simulink model "IEEE14_case"  (R2024b)
settings: Solver=FixedStepAuto  StartTime=0  StopTime=2  FixedStep=1e-7  RelTol=1e-3
values from neighbouring files (symbols this model uses):
  GFL_15_Bva = 0.009    [IEEE14_parameters.m]
  GFL_15_C_bus_pu = 7.179419    [IEEE14_parameters.m]
  GFL_15_f0 = 60    [IEEE14_parameters.m]
  GFL_15_I_id = 691.26967    [IEEE14_parameters.m]
  GFL_15_I_iq = 691.26967    [IEEE14_parameters.m]
  GFL_15_I_od = 45.2207    [IEEE14_parameters.m]
  GFL_15_I_oq = 45.2207    [IEEE14_parameters.m]
  GFL_15_I_pll = 0.78    [IEEE14_parameters.m]
  GFL_15_Kdi = 0.09    [IEEE14_parameters.m]
  GFL_15_Kdo = 0.9    [IEEE14_parameters.m]
  GFL_15_Kqi = 0.09    [IEEE14_parameters.m]
  GFL_15_Kqo = 0.9    [IEEE14_parameters.m]
  GFL_15_Lg_pu = 0.631447    [IEEE14_parameters.m]
  GFL_15_mode = 1    [IEEE14_parameters.m]
  GFL_15_P_id = 3.7166    [IEEE14_parameters.m]
  GFL_15_P_iq = 3.7166    [IEEE14_parameters.m]
  GFL_15_P_od = 0.4798    [IEEE14_parameters.m]
  GFL_15_P_oq = 0.4798    [IEEE14_parameters.m]
  GFL_15_P_pll = 290.42    [IEEE14_parameters.m]
  GFL_15_Qe_ref = 0.2    [IEEE14_parameters.m]
  GFL_15_Rg_pu = 0.024016    [IEEE14_parameters.m]
  GFL_15_Sbase = 1.000000e+4    (= 10000)    [IEEE14_parameters.m]
  GFL_15_Tdi = 0.01    [IEEE14_parameters.m]
  GFL_15_Tdo = 0.2    [IEEE14_parameters.m]
  GFL_15_Tqi = 0.01    [IEEE14_parameters.m]
  GFL_15_Tqo = 0.2    [IEEE14_parameters.m]
  GFL_15_Vbase = 380    [IEEE14_parameters.m]
  GFL_15_Vdc_ref = 1.011475    [IEEE14_parameters.m]
  GFL_15_Vdcbase = 700    [IEEE14_parameters.m]
  GFL_15_vq_ref = 0    [IEEE14_parameters.m]
  GFL_16_Bva = 0.002    [IEEE14_parameters.m]
  GFL_16_C_bus_pu = 7.179419    [IEEE14_parameters.m]
  GFL_16_f0 = 60    [IEEE14_parameters.m]
  GFL_16_I_id = 691.26967    [IEEE14_parameters.m]
  GFL_16_I_iq = 691.26967    [IEEE14_parameters.m]
  GFL_16_I_od = 45.2207    [IEEE14_parameters.m]
  GFL_16_I_oq = 45.2207    [IEEE14_parameters.m]
  GFL_16_I_pll = 0.78    [IEEE14_parameters.m]
  GFL_16_Kdi = 0.05    [IEEE14_parameters.m]
  GFL_16_Kdo = 0.5    [IEEE14_parameters.m]
  GFL_16_Kqi = 0.05    [IEEE14_parameters.m]
  GFL_16_Kqo = 0.5    [IEEE14_parameters.m]
  GFL_16_Lg_pu = 0.631447    [IEEE14_parameters.m]
  GFL_16_mode = 1    [IEEE14_parameters.m]
  GFL_16_P_id = 3.7166    [IEEE14_parameters.m]
  GFL_16_P_iq = 3.7166    [IEEE14_parameters.m]
  GFL_16_P_od = 0.4798    [IEEE14_parameters.m]
  GFL_16_P_oq = 0.4798    [IEEE14_parameters.m]
  GFL_16_P_pll = 290.42    [IEEE14_parameters.m]
  GFL_16_Qe_ref = 0.2    [IEEE14_parameters.m]
  GFL_16_Rg_pu = 0.024016    [IEEE14_parameters.m]
  GFL_16_Sbase = 1.000000e+4    (= 10000)    [IEEE14_parameters.m]
  GFL_16_Tdi = 0.01    [IEEE14_parameters.m]
  GFL_16_Tdo = 0.2    [IEEE14_parameters.m]
  GFL_16_Tqi = 0.01    [IEEE14_parameters.m]
  GFL_16_Tqo = 0.2    [IEEE14_parameters.m]
  GFL_16_Vbase = 380    [IEEE14_parameters.m]
  GFL_16_Vdc_ref = 1.01144    [IEEE14_parameters.m]
  GFL_16_Vdcbase = 700    [IEEE14_parameters.m]
  GFL_16_vq_ref = 0    [IEEE14_parameters.m]
  GFL_17_Bva = 0.002    [IEEE14_parameters.m]
  GFL_17_C_bus_pu = 7.179419    [IEEE14_parameters.m]
  GFL_17_f0 = 60    [IEEE14_parameters.m]
  GFL_17_I_id = 691.26967    [IEEE14_parameters.m]
  GFL_17_I_iq = 691.26967    [IEEE14_parameters.m]
  GFL_17_I_od = 45.2207    [IEEE14_parameters.m]
  GFL_17_I_oq = 45.2207    [IEEE14_parameters.m]
  GFL_17_I_pll = 0.78    [IEEE14_parameters.m]
  GFL_17_Kdi = 0.05    [IEEE14_parameters.m]
  GFL_17_Kdo = 0.5    [IEEE14_parameters.m]
  GFL_17_Kqi = 0.05    [IEEE14_parameters.m]
  GFL_17_Kqo = 0.5    [IEEE14_parameters.m]
  GFL_17_Lg_pu = 0.631447    [IEEE14_parameters.m]
  GFL_17_mode = 1    [IEEE14_parameters.m]
  GFL_17_P_id = 3.7166    [IEEE14_parameters.m]
  GFL_17_P_iq = 3.7166    [IEEE14_parameters.m]
  GFL_17_P_od = 0.4798    [IEEE14_parameters.m]
  GFL_17_P_oq = 0.4798    [IEEE14_parameters.m]
  GFL_17_P_pll = 290.42    [IEEE14_parameters.m]
  GFL_17_Qe_ref = 0.2    [IEEE14_parameters.m]
  GFL_17_Rg_pu = 0.024016    [IEEE14_parameters.m]
  GFL_17_Sbase = 1.000000e+4    (= 10000)    [IEEE14_parameters.m]
  GFL_17_Tdi = 0.01    [IEEE14_parameters.m]
  GFL_17_Tdo = 0.2    [IEEE14_parameters.m]
  GFL_17_Tqi = 0.01    [IEEE14_parameters.m]
  GFL_17_Tqo = 0.2    [IEEE14_parameters.m]
  GFL_17_Vbase = 380    [IEEE14_parameters.m]
  GFL_17_Vdc_ref = 1.011632    [IEEE14_parameters.m]
  GFL_17_Vdcbase = 700    [IEEE14_parameters.m]
  GFL_17_vq_ref = 0    [IEEE14_parameters.m]
  GFL_18_Bva = 0.002    [IEEE14_parameters.m]
  GFL_18_C_bus_pu = 7.179419    [IEEE14_parameters.m]
  GFL_18_f0 = 60    [IEEE14_parameters.m]
  GFL_18_I_id = 691.26967    [IEEE14_parameters.m]
  GFL_18_I_iq = 691.26967    [IEEE14_parameters.m]
  GFL_18_I_od = 45.2207    [IEEE14_parameters.m]
  GFL_18_I_oq = 45.2207    [IEEE14_parameters.m]
  GFL_18_I_pll = 0.78    [IEEE14_parameters.m]
  GFL_18_Kdi = 0.05    [IEEE14_parameters.m]
  GFL_18_Kdo = 0.5    [IEEE14_parameters.m]
  GFL_18_Kqi = 0.05    [IEEE14_parameters.m]
  GFL_18_Kqo = 0.5    [IEEE14_parameters.m]
  GFL_18_Lg_pu = 0.631447    [IEEE14_parameters.m]
  GFL_18_mode = 1    [IEEE14_parameters.m]
  GFL_18_P_id = 3.7166    [IEEE14_parameters.m]
  GFL_18_P_iq = 3.7166    [IEEE14_parameters.m]
  GFL_18_P_od = 0.4798    [IEEE14_parameters.m]
  GFL_18_P_oq = 0.4798    [IEEE14_parameters.m]
  GFL_18_P_pll = 290.42    [IEEE14_parameters.m]
  GFL_18_Qe_ref = 0.2    [IEEE14_parameters.m]
  GFL_18_Rg_pu = 0.024016    [IEEE14_parameters.m]
  GFL_18_Sbase = 1.000000e+4    (= 10000)    [IEEE14_parameters.m]
  GFL_18_Tdi = 0.01    [IEEE14_parameters.m]
  GFL_18_Tdo = 0.2    [IEEE14_parameters.m]
  GFL_18_Tqi = 0.01    [IEEE14_parameters.m]
  GFL_18_Tqo = 0.2    [IEEE14_parameters.m]
  GFL_18_Vbase = 380    [IEEE14_parameters.m]
  GFL_18_Vdc_ref = 1.011572    [IEEE14_parameters.m]
  GFL_18_Vdcbase = 700    [IEEE14_parameters.m]
  GFL_18_vq_ref = 0    [IEEE14_parameters.m]
  ... (+180 more)
(part 3 of 25)

== system IEEE14_case/GFL_15 ==
  v_d_GFL_15 : Inport
  v_q_GFL_15 : Inport  Port=2
  i_dc_GFL_15 : Inport  Port=3
  Idv_GFL_15 : Integrator  InitialCondition=-9.005176619289375e-21
  Iqv_GFL_15 : Integrator  InitialCondition=212.99246240000113
  Phi_ga_GFL_15 : Integrator  InitialCondition=14.405272691494698
  Phi_gb_GFL_15 : Integrator  InitialCondition=4.700156753170725
  Phi_gc_GFL_15 : Integrator  InitialCondition=-215.7031229683803
  Phi_gd_GFL_15 : Integrator  InitialCondition=-0.9400313506342463
  Phipll_GFL_15 : Integrator  InitialCondition=-8.990901410054388e-21
  Psi_d_GFL_15 : Integrator  InitialCondition=1.758329914032016e-21
  Psi_q_GFL_15 : Integrator  InitialCondition=21.299246240000112
  V_dc_GFL_15 : Integrator  InitialCondition=708.0324770006274
  d_Idv_GFL_15_block : Subsystem
  d_Iqv_GFL_15_block : Subsystem
  d_Phi_ga_GFL_15_block : Subsystem
  d_Phi_gb_GFL_15_block : Subsystem
  d_Phi_gc_GFL_15_block : Subsystem
  d_Phi_gd_GFL_15_block : Subsystem
  d_Phipll_GFL_15_block : Subsystem
  d_Psi_d_GFL_15_block : Subsystem
  d_Psi_q_GFL_15_block : Subsystem
  d_V_dc_GFL_15_block : Subsystem
  d_i_gd_GFL_15_block : Subsystem
  d_i_gq_GFL_15_block : Subsystem
  d_theta_pll_GFL_15_block : Subsystem
  e_dc_GFL_15_block : Subsystem
  i_d_GFL_15_block : Subsystem
  i_gd_GFL_15 : Integrator  InitialCondition=13.553302841894695
  i_gq_GFL_15 : Integrator  InitialCondition=-2.710660568379226
  i_q_GFL_15_block : Subsystem
  theta_pll_GFL_15 : Integrator  InitialCondition=0.12960466832124
  i_d_GFL_15 : Outport
  i_q_GFL_15 : Outport  Port=2
  e_dc_GFL_15 : Outport  Port=3
  wires:
  V_dc_GFL_15/1 -> d_V_dc_GFL_15_block/1(State_V_dc_GFL_15_d284c), d_V_dc_GFL_15_block/10(State_V_dc_GFL_15_e0213), d_V_dc_GFL_15_block/42(State_V_dc_GFL_15_5df59), d_i_gd_GFL_15_block/6(State_V_dc_GFL_15_5ead9), d_Phi_gb_GFL_15_block/6(State_V_dc_GFL_15_cf545), d_Phi_ga_GFL_15_block/1(State_V_dc_GFL_15_371a8), e_dc_GFL_15_block/1(State_V_dc_GFL_15_93b67)
  theta_pll_GFL_15/1 -> d_i_gq_GFL_15_block/10(State_theta_pll_GFL_15_ed7e5), d_i_gq_GFL_15_block/13(State_theta_pll_GFL_15_a894f), d_i_gq_GFL_15_block/15(State_theta_pll_GFL_15_7b0e7), d_V_dc_GFL_15_block/6(State_theta_pll_GFL_15_67f5c), d_i_gq_GFL_15_block/8(State_theta_pll_GFL_15_b231d), d_V_dc_GFL_15_block/8(State_theta_pll_GFL_15_bdd37), d_V_dc_GFL_15_block/15(State_theta_pll_GFL_15_3bef8), d_V_dc_GFL_15_block/17(State_theta_pll_GFL_15_b898b), d_V_dc_GFL_15_block/23(State_theta_pll_GFL_15_82eb1), d_V_dc_GFL_15_block/27(State_theta_pll_GFL_15_9ca51), d_V_dc_GFL_15_block/32(State_theta_pll_GFL_15_ec66b), d_i_gd_GFL_15_block/4(State_theta_pll_GFL_15_781ce), d_V_dc_GFL_15_block/34(State_theta_pll_GFL_15_4b302), d_i_gq_GFL_15_block/2(State_theta_pll_GFL_15_94dd7), d_V_dc_GFL_15_block/41(State_theta_pll_GFL_15_0f1b8), d_theta_pll_GFL_15_block/4(State_theta_pll_GFL_15_f7355), d_Phi_gb_GFL_15_block/2(State_theta_pll_GFL_15_82324), d_Phi_gb_GFL_15_block/4(State_theta_pll_GFL_15_58522), d_V_dc_GFL_15_block/39(State_theta_pll_GFL_15_39e34), d_Phi_gd_GFL_15_block/4(State_theta_pll_GFL_15_d2b83), d_Phi_gd_GFL_15_block/2(State_theta_pll_GFL_15_e398b), d_Phi_gd_GFL_15_block/8(State_theta_pll_GFL_15_37f0e), d_Phi_gd_GFL_15_block/10(State_theta_pll_GFL_15_ae580), d_Phi_gd_GFL_15_block/13(State_theta_pll_GFL_15_e05ad), d_Phi_gd_GFL_15_block/15(State_theta_pll_GFL_15_0e420), d_Idv_GFL_15_block/3(State_theta_pll_GFL_15_12ffd), d_Idv_GFL_15_block/5(State_theta_pll_GFL_15_9725f), d_i_gq_GFL_15_block/4(State_theta_pll_GFL_15_89960), d_Idv_GFL_15_block/9(State_theta_pll_GFL_15_2202b), d_Iqv_GFL_15_block/9(State_theta_pll_GFL_15_f624d), d_V_dc_GFL_15_block/21(State_theta_pll_GFL_15_c9fe8), d_Iqv_GFL_15_block/7(State_theta_pll_GFL_15_e8e0d), d_Iqv_GFL_15_block/3(State_theta_pll_GFL_15_5bce6), d_i_gd_GFL_15_block/2(State_theta_pll_GFL_15_a07ec), d_Iqv_GFL_15_block/5(State_theta_pll_GFL_15_c6881), d_Phipll_GFL_15_block/2(State_theta_pll_GFL_15_65253), d_Phi_gc_GFL_15_block/3(State_theta_pll_GFL_15_5b93f), d_Phi_gc_GFL_15_block/5(State_theta_pll_GFL_15_647bc), d_Phi_gc_GFL_15_block/10(State_theta_pll_GFL_15_159ad), d_Psi_d_GFL_15_block/2(State_theta_pll_GFL_15_95588), d_Psi_d_GFL_15_block/4(State_theta_pll_GFL_15_90724), d_Psi_q_GFL_15_block/2(State_theta_pll_GFL_15_42098), d_Psi_q_GFL_15_block/4(State_theta_pll_GFL_15_5b172), i_d_GFL_15_block/2(State_theta_pll_GFL_15_42e0c), i_d_GFL_15_block/4(State_theta_pll_GFL_15_0eec4), i_q_GFL_15_block/2(State_theta_pll_GFL_15_f2c21), i_q_GFL_15_block/4(State_theta_pll_GFL_15_a18db), d_Phi_gc_GFL_15_block/8(State_theta_pll_GFL_15_01aaa), d_Phipll_GFL_15_block/4(State_theta_pll_GFL_15_facf8), d_Idv_GFL_15_block/7(State_theta_pll_GFL_15_963fe), d_V_dc_GFL_15_block/29(State_theta_pll_GFL_15_fe7b4), d_theta_pll_GFL_15_block/2(State_theta_pll_GFL_15_a4865)
  Phipll_GFL_15/1 -> d_theta_pll_GFL_15_block/5(State_Phipll_GFL_15_52c7d)
  v_q_GFL_15/1 -> d_i_gq_GFL_15_block/9(Input_v_q_GFL_15_75f43), d_V_dc_GFL_15_block/7(Input_v_q_GFL_15_c44d2), d_V_dc_GFL_15_block/16(Input_v_q_GFL_15_c31da), d_V_dc_GFL_15_block/22(Input_v_q_GFL_15_2238e), d_V_dc_GFL_15_block/28(Input_v_q_GFL_15_ed91f), d_V_dc_GFL_15_block/33(Input_v_q_GFL_15_9b8d9), d_Phi_gb_GFL_15_block/3(Input_v_q_GFL_15_e2248), d_Phi_gd_GFL_15_block/3(Input_v_q_GFL_15_9f181), d_Phi_gd_GFL_15_block/9(Input_v_q_GFL_15_fe173), d_Phi_gd_GFL_15_block/14(Input_v_q_GFL_15_7c25a), d_Idv_GFL_15_block/4(Input_v_q_GFL_15_617c4), d_Idv_GFL_15_block/8(Input_v_q_GFL_15_86e6c), d_Iqv_GFL_15_block/4(Input_v_q_GFL_15_4a34b), d_i_gd_GFL_15_block/3(Input_v_q_GFL_15_bfddf), d_i_gq_GFL_15_block/14(Input_v_q_GFL_15_7f556), d_V_dc_GFL_15_block/40(Input_v_q_GFL_15_f41a7), d_Iqv_GFL_15_block/8(Input_v_q_GFL_15_924af), d_theta_pll_GFL_15_block/3(Input_v_q_GFL_15_7e43d), d_i_gq_GFL_15_block/3(Input_v_q_GFL_15_1b267), d_Phipll_GFL_15_block/3(Input_v_q_GFL_15_2a56a), d_Phi_gc_GFL_15_block/4(Input_v_q_GFL_15_7ae45), d_Phi_gc_GFL_15_block/9(Input_v_q_GFL_15_e532d), d_Psi_d_GFL_15_block/3(Input_v_q_GFL_15_84d7e), d_Psi_q_GFL_15_block/3(Input_v_q_GFL_15_da40e)
  i_dc_GFL_15/1 -> d_V_dc_GFL_15_block/2(Input_i_dc_GFL_15_d0365)
  d_Iqv_GFL_15_block/1(Blockout_d_Iqv_GFL_15_65918) -> Iqv_GFL_15/1
  d_i_gq_GFL_15_block/1(Blockout_d_i_gq_GFL_15_fa7d1) -> i_gq_GFL_15/1
  d_Psi_d_GFL_15_block/1(Blockout_d_Psi_d_GFL_15_bd2bd) -> Psi_d_GFL_15/1
  d_Idv_GFL_15_block/1(Blockout_d_Idv_GFL_15_06d8e) -> Idv_GFL_15/1
  e_dc_GFL_15_block/1(Blockout_e_dc_GFL_15_d58b9) -> e_dc_GFL_15/1
  Psi_d_GFL_15/1 -> d_Psi_d_GFL_15_block/5(State_Psi_d_GFL_15_90def), d_Idv_GFL_15_block/10(State_Psi_d_GFL_15_22a12)
  i_q_GFL_15_block/1(Blockout_i_q_GFL_15_86262) -> i_q_GFL_15/1
  Idv_GFL_15/1 -> d_V_dc_GFL_15_block/9(State_Idv_GFL_15_d358d), d_Idv_GFL_15_block/1(State_Idv_GFL_15_ca6d1), d_i_gd_GFL_15_block/5(State_Idv_GFL_15_0b38b), d_Phi_gb_GFL_15_block/5(State_Idv_GFL_15_4c70c)
  Iqv_GFL_15/1 -> d_Iqv_GFL_15_block/1(State_Iqv_GFL_15_a0efa), d_V_dc_GFL_15_block/24(State_Iqv_GFL_15_f2022), d_i_gq_GFL_15_block/5(State_Iqv_GFL_15_5d544), d_Phi_gd_GFL_15_block/5(State_Iqv_GFL_15_f6823)
  i_d_GFL_15_block/1(Blockout_i_d_GFL_15_9798a) -> i_d_GFL_15/1
  d_Phipll_GFL_15_block/1(Blockout_d_Phipll_GFL_15_2e0e5) -> Phipll_GFL_15/1
  d_Psi_q_GFL_15_block/1(Blockout_d_Psi_q_GFL_15_d79bb) -> Psi_q_GFL_15/1
  d_Phi_gd_GFL_15_block/1(Blockout_d_Phi_gd_GFL_15_84e3d) -> Phi_gd_GFL_15/1
  d_Phi_gc_GFL_15_block/1(Blockout_d_Phi_gc_GFL_15_8e044) -> Phi_gc_GFL_15/1
  d_Phi_gb_GFL_15_block/1(Blockout_d_Phi_gb_GFL_15_f24ee) -> Phi_gb_GFL_15/1
  i_gd_GFL_15/1 -> d_i_gd_GFL_15_block/10(State_i_gd_GFL_15_48775), d_i_gq_GFL_15_block/6(State_i_gd_GFL_15_18b61), d_V_dc_GFL_15_block/3(State_i_gd_GFL_15_cdb92), d_V_dc_GFL_15_block/12(State_i_gd_GFL_15_079b9), d_Phi_gd_GFL_15_block/6(State_i_gd_GFL_15_7f54c), d_Phi_gb_GFL_15_block/8(State_i_gd_GFL_15_ca8ed), d_i_gd_GFL_15_block/8(State_i_gd_GFL_15_d802d), d_V_dc_GFL_15_block/25(State_i_gd_GFL_15_6b04f), i_d_GFL_15_block/1(State_i_gd_GFL_15_2eb7d), i_q_GFL_15_block/1(State_i_gd_GFL_15_ae75b), d_V_dc_GFL_15_block/19(State_i_gd_GFL_15_14a00), d_Phi_gc_GFL_15_block/1(State_i_gd_GFL_15_68d30)
  d_Phi_ga_GFL_15_block/1(Blockout_d_Phi_ga_GFL_15_ed294) -> Phi_ga_GFL_15/1
  d_V_dc_GFL_15_block/1(Blockout_d_V_dc_GFL_15_869f2) -> V_dc_GFL_15/1
  Phi_gc_GFL_15/1 -> d_i_gq_GFL_15_block/16(State_Phi_gc_GFL_15_ddb2f), d_Phi_gd_GFL_15_block/16(State_Phi_gc_GFL_15_d40bd), d_V_dc_GFL_15_block/35(State_Phi_gc_GFL_15_695ea)
  Phi_gd_GFL_15/1 -> d_V_dc_GFL_15_block/37(State_Phi_gd_GFL_15_85b08), d_i_gq_GFL_15_block/18(State_Phi_gd_GFL_15_8521d)
  d_i_gd_GFL_15_block/1(Blockout_d_i_gd_GFL_15_2c157) -> i_gd_GFL_15/1
  Psi_q_GFL_15/1 -> d_Psi_q_GFL_15_block/5(State_Psi_q_GFL_15_c1e2a), d_Iqv_GFL_15_block/10(State_Psi_q_GFL_15_d75c1)
  i_gq_GFL_15/1 -> d_V_dc_GFL_15_block/4(State_i_gq_GFL_15_e301f), d_V_dc_GFL_15_block/18(State_i_gq_GFL_15_6885c), d_Phi_gd_GFL_15_block/11(State_i_gq_GFL_15_08dfd), d_i_gq_GFL_15_block/17(State_i_gq_GFL_15_84adb), d_i_gq_GFL_15_block/11(State_i_gq_GFL_15_b1e74), d_Phi_gd_GFL_15_block/17(State_i_gq_GFL_15_39259), d_V_dc_GFL_15_block/30(State_i_gq_GFL_15_2eb02), d_i_gq_GFL_15_block/19(State_i_gq_GFL_15_e4e41), d_Phi_gc_GFL_15_block/6(State_i_gq_GFL_15_2aff2), i_d_GFL_15_block/3(State_i_gq_GFL_15_49ce8), i_q_GFL_15_block/3(State_i_gq_GFL_15_dea28), d_V_dc_GFL_15_block/36(State_i_gq_GFL_15_5f189)
  Phi_gb_GFL_15/1 -> d_V_dc_GFL_15_block/13(State_Phi_gb_GFL_15_4966d), d_i_gd_GFL_15_block/9(State_Phi_gb_GFL_15_ef282)
  Phi_ga_GFL_15/1 -> d_V_dc_GFL_15_block/11(State_Phi_ga_GFL_15_78944), d_i_gd_GFL_15_block/7(State_Phi_ga_GFL_15_6d748), d_Phi_gb_GFL_15_block/7(State_Phi_ga_GFL_15_778c9)
  v_d_GFL_15/1 -> d_i_gd_GFL_15_block/1(Input_v_d_GFL_15_1fa3a), d_i_gq_GFL_15_block/1(Input_v_d_GFL_15_d1f59), d_i_gq_GFL_15_block/7(Input_v_d_GFL_15_8be69), d_i_gq_GFL_15_block/12(Input_v_d_GFL_15_06aad), d_V_dc_GFL_15_block/5(Input_v_d_GFL_15_4e2a8), d_V_dc_GFL_15_block/14(Input_v_d_GFL_15_eebae), d_V_dc_GFL_15_block/20(Input_v_d_GFL_15_9f0d6), d_V_dc_GFL_15_block/31(Input_v_d_GFL_15_991b5), d_V_dc_GFL_15_block/26(Input_v_d_GFL_15_3ac4b), d_V_dc_GFL_15_block/38(Input_v_d_GFL_15_ab6c9), d_theta_pll_GFL_15_block/1(Input_v_d_GFL_15_6336d), d_Phi_gd_GFL_15_block/12(Input_v_d_GFL_15_96988), d_Phi_gb_GFL_15_block/1(Input_v_d_GFL_15_ba16a), d_Phi_gd_GFL_15_block/7(Input_v_d_GFL_15_19381), d_Idv_GFL_15_block/2(Input_v_d_GFL_15_d6ef0), d_Phi_gd_GFL_15_block/1(Input_v_d_GFL_15_e0c96), d_Idv_GFL_15_block/6(Input_v_d_GFL_15_adaa4), d_Iqv_GFL_15_block/2(Input_v_d_GFL_15_e9447), d_Iqv_GFL_15_block/6(Input_v_d_GFL_15_7c93a), d_Phipll_GFL_15_block/1(Input_v_d_GFL_15_62a1f), d_Phi_gc_GFL_15_block/2(Input_v_d_GFL_15_05f07), d_Phi_gc_GFL_15_block/7(Input_v_d_GFL_15_b97ec), d_Psi_d_GFL_15_block/1(Input_v_d_GFL_15_d26c2), d_Psi_q_GFL_15_block/1(Input_v_d_GFL_15_07bda)
  d_theta_pll_GFL_15_block/1(Blockout_d_theta_pll_GFL_15_bcede) -> theta_pll_GFL_15/1

== system IEEE14_case/GFL_16 ==
  v_d_GFL_16 : Inport
  v_q_GFL_16 : Inport  Port=2
  i_dc_GFL_16 : Inport  Port=3
  Idv_GFL_16 : Integrator  InitialCondition=-3.057046097222704e-20
  Iqv_GFL_16 : Integrator  InitialCondition=213.31675440000038
  Phi_ga_GFL_16 : Integrator  InitialCondition=14.385965628488423
  Phi_gb_GFL_16 : Integrator  InitialCondition=4.69301140147029
  Phi_gc_GFL_16 : Integrator  InitialCondition=-216.02329412217819
  Phi_gd_GFL_16 : Integrator  InitialCondition=-0.9386022802940988
  Phipll_GFL_16 : Integrator  InitialCondition=7.7116362328713e-21
  Psi_d_GFL_16 : Integrator  InitialCondition=1.3342711491415958e-22
  Psi_q_GFL_16 : Integrator  InitialCondition=21.33167544000004
  V_dc_GFL_16 : Integrator  InitialCondition=708.0080730370232
  d_Idv_GFL_16_block : Subsystem
  d_Iqv_GFL_16_block : Subsystem
  d_Phi_ga_GFL_16_block : Subsystem
  d_Phi_gb_GFL_16_block : Subsystem
  d_Phi_gc_GFL_16_block : Subsystem
  d_Phi_gd_GFL_16_block : Subsystem
  d_Phipll_GFL_16_block : Subsystem
  d_Psi_d_GFL_16_block : Subsystem
  d_Psi_q_GFL_16_block : Subsystem
  d_V_dc_GFL_16_block : Subsystem
  d_i_gd_GFL_16_block : Subsystem
  d_i_gq_GFL_16_block : Subsystem
  d_theta_pll_GFL_16_block : Subsystem
  e_dc_GFL_16_block : Subsystem
  i_d_GFL_16_block : Subsystem
  i_gd_GFL_16 : Integrator  InitialCondition=13.53269861088842
  i_gq_GFL_16 : Integrator  InitialCondition=-2.7065397221778023
  i_q_GFL_16_block : Subsystem
  theta_pll_GFL_16 : Integrator  InitialCondition=0.12416858554783365
  i_d_GFL_16 : Outport
  i_q_GFL_16 : Outport  Port=2
  e_dc_GFL_16 : Outport  Port=3
  wires:
  V_dc_GFL_16/1 -> d_V_dc_GFL_16_block/42(State_V_dc_GFL_16_a6d1b), d_V_dc_GFL_16_block/1(State_V_dc_GFL_16_d7b7a), d_V_dc_GFL_16_block/10(State_V_dc_GFL_16_5e24a), d_i_gd_GFL_16_block/6(State_V_dc_GFL_16_82701), d_Phi_gb_GFL_16_block/6(State_V_dc_GFL_16_186eb), d_Phi_ga_GFL_16_block/1(State_V_dc_GFL_16_db5ba), e_dc_GFL_16_block/1(State_V_dc_GFL_16_ba6ae)
  Phipll_GFL_16/1 -> d_theta_pll_GFL_16_block/5(State_Phipll_GFL_16_9e2b9)
  e_dc_GFL_16_block/1(Blockout_e_dc_GFL_16_30897) -> e_dc_GFL_16/1
  i_dc_GFL_16/1 -> d_V_dc_GFL_16_block/2(Input_i_dc_GFL_16_33564)
  d_theta_pll_GFL_16_block/1(Blockout_d_theta_pll_GFL_16_374a4) -> theta_pll_GFL_16/1
  d_Psi_q_GFL_16_block/1(Blockout_d_Psi_q_GFL_16_c83e3) -> Psi_q_GFL_16/1
  d_Idv_GFL_16_block/1(Blockout_d_Idv_GFL_16_0d833) -> Idv_GFL_16/1
  d_Psi_d_GFL_16_block/1(Blockout_d_Psi_d_GFL_16_a9046) -> Psi_d_GFL_16/1
  i_gd_GFL_16/1 -> d_i_gd_GFL_16_block/10(State_i_gd_GFL_16_5edc7), d_i_gq_GFL_16_block/6(State_i_gd_GFL_16_461cd), d_Phi_gb_GFL_16_block/8(State_i_gd_GFL_16_104f5), d_V_dc_GFL_16_block/3(State_i_gd_GFL_16_cdb96), d_V_dc_GFL_16_block/19(State_i_gd_GFL_16_d36c8), d_i_gd_GFL_16_block/8(State_i_gd_GFL_16_54b5c), d_V_dc_GFL_16_block/25(State_i_gd_GFL_16_27e02), d_Phi_gd_GFL_16_block/6(State_i_gd_GFL_16_6aeee), d_V_dc_GFL_16_block/12(State_i_gd_GFL_16_d2743), i_d_GFL_16_block/1(State_i_gd_GFL_16_f9181), d_Phi_gc_GFL_16_block/1(State_i_gd_GFL_16_f5bc3), i_q_GFL_16_block/1(State_i_gd_GFL_16_ab236)
  Phi_ga_GFL_16/1 -> d_V_dc_GFL_16_block/11(State_Phi_ga_GFL_16_f5490), d_i_gd_GFL_16_block/7(State_Phi_ga_GFL_16_0916f), d_Phi_gb_GFL_16_block/7(State_Phi_ga_GFL_16_9aa12)
  Phi_gd_GFL_16/1 -> d_V_dc_GFL_16_block/37(State_Phi_gd_GFL_16_9eb81), d_i_gq_GFL_16_block/18(State_Phi_gd_GFL_16_6ff49)
  i_q_GFL_16_block/1(Blockout_i_q_GFL_16_30f67) -> i_q_GFL_16/1
  d_Iqv_GFL_16_block/1(Blockout_d_Iqv_GFL_16_b60c7) -> Iqv_GFL_16/1
  d_i_gq_GFL_16_block/1(Blockout_d_i_gq_GFL_16_4ea9b) -> i_gq_GFL_16/1
  Idv_GFL_16/1 -> d_V_dc_GFL_16_block/9(State_Idv_GFL_16_247ed), d_Idv_GFL_16_block/1(State_Idv_GFL_16_21a9b), d_Phi_gb_GFL_16_block/5(State_Idv_GFL_16_00ce2), d_i_gd_GFL_16_block/5(State_Idv_GFL_16_f06d3)
  d_i_gd_GFL_16_block/1(Blockout_d_i_gd_GFL_16_c534c) -> i_gd_GFL_16/1
  Psi_q_GFL_16/1 -> d_Psi_q_GFL_16_block/5(State_Psi_q_GFL_16_7f6e6), d_Iqv_GFL_16_block/10(State_Psi_q_GFL_16_4f61f)
  i_gq_GFL_16/1 -> d_V_dc_GFL_16_block/4(State_i_gq_GFL_16_0cd26), d_V_dc_GFL_16_block/30(State_i_gq_GFL_16_bf6cb), d_Phi_gd_GFL_16_block/17(State_i_gq_GFL_16_a143d), d_Phi_gd_GFL_16_block/11(State_i_gq_GFL_16_a69ee), d_V_dc_GFL_16_block/18(State_i_gq_GFL_16_94bfe), d_i_gq_GFL_16_block/19(State_i_gq_GFL_16_bb299), d_i_gq_GFL_16_block/11(State_i_gq_GFL_16_8af0d), d_V_dc_GFL_16_block/36(State_i_gq_GFL_16_76021), d_i_gq_GFL_16_block/17(State_i_gq_GFL_16_f0d16), d_Phi_gc_GFL_16_block/6(State_i_gq_GFL_16_12809), i_d_GFL_16_block/3(State_i_gq_GFL_16_5d9af), i_q_GFL_16_block/3(State_i_gq_GFL_16_367d1)
  i_d_GFL_16_block/1(Blockout_i_d_GFL_16_cb76b) -> i_d_GFL_16/1
  d_Phi_gd_GFL_16_block/1(Blockout_d_Phi_gd_GFL_16_8a731) -> Phi_gd_GFL_16/1
  theta_pll_GFL_16/1 -> d_i_gd_GFL_16_block/4(State_theta_pll_GFL_16_7ef19), d_i_gq_GFL_16_block/4(State_theta_pll_GFL_16_3325f), d_i_gq_GFL_16_block/8(State_theta_pll_GFL_16_b6938), d_i_gq_GFL_16_block/13(State_theta_pll_GFL_16_f68d0), d_V_dc_GFL_16_block/15(State_theta_pll_GFL_16_c4182), d_V_dc_GFL_16_block/21(State_theta_pll_GFL_16_9aada), d_V_dc_GFL_16_block/27(State_theta_pll_GFL_16_b1199), d_V_dc_GFL_16_block/29(State_theta_pll_GFL_16_7f4e3), d_V_dc_GFL_16_block/6(State_theta_pll_GFL_16_59dfe), d_V_dc_GFL_16_block/41(State_theta_pll_GFL_16_36915), d_V_dc_GFL_16_block/39(State_theta_pll_GFL_16_5537f), d_V_dc_GFL_16_block/8(State_theta_pll_GFL_16_4472e), d_theta_pll_GFL_16_block/2(State_theta_pll_GFL_16_60b13), d_i_gq_GFL_16_block/2(State_theta_pll_GFL_16_b9b0c), d_theta_pll_GFL_16_block/4(State_theta_pll_GFL_16_eb390), d_V_dc_GFL_16_block/34(State_theta_pll_GFL_16_c3157), d_Phi_gb_GFL_16_block/4(State_theta_pll_GFL_16_1f0e5), d_Phi_gd_GFL_16_block/2(State_theta_pll_GFL_16_648b2), d_Phi_gd_GFL_16_block/4(State_theta_pll_GFL_16_e1421), d_Phi_gd_GFL_16_block/13(State_theta_pll_GFL_16_6f123), d_Phi_gd_GFL_16_block/15(State_theta_pll_GFL_16_ebd89), d_Phi_gd_GFL_16_block/8(State_theta_pll_GFL_16_9c942), d_Idv_GFL_16_block/3(State_theta_pll_GFL_16_5434c), d_Idv_GFL_16_block/7(State_theta_pll_GFL_16_d4b0d), d_Phi_gd_GFL_16_block/10(State_theta_pll_GFL_16_5c378), d_Iqv_GFL_16_block/3(State_theta_pll_GFL_16_74ff7), d_Iqv_GFL_16_block/7(State_theta_pll_GFL_16_5893a), d_Iqv_GFL_16_block/5(State_theta_pll_GFL_16_ecda2), d_V_dc_GFL_16_block/17(State_theta_pll_GFL_16_f0853), d_Idv_GFL_16_block/5(State_theta_pll_GFL_16_fe8ca), d_V_dc_GFL_16_block/23(State_theta_pll_GFL_16_8b441), d_i_gq_GFL_16_block/15(State_theta_pll_GFL_16_2ae3b), d_i_gd_GFL_16_block/2(State_theta_pll_GFL_16_0c1ff), d_Phi_gb_GFL_16_block/2(State_theta_pll_GFL_16_9faca), d_i_gq_GFL_16_block/10(State_theta_pll_GFL_16_ce5b5), d_Phipll_GFL_16_block/4(State_theta_pll_GFL_16_5a7c5), d_Phi_gc_GFL_16_block/5(State_theta_pll_GFL_16_9a1c0), d_Phi_gc_GFL_16_block/8(State_theta_pll_GFL_16_c56ef), d_Phi_gc_GFL_16_block/10(State_theta_pll_GFL_16_a6854), d_V_dc_GFL_16_block/32(State_theta_pll_GFL_16_e0209), d_Psi_d_GFL_16_block/4(State_theta_pll_GFL_16_41daa), d_Psi_q_GFL_16_block/2(State_theta_pll_GFL_16_b008b), d_Psi_q_GFL_16_block/4(State_theta_pll_GFL_16_07f68), d_Phi_gc_GFL_16_block/3(State_theta_pll_GFL_16_2a2ae), i_q_GFL_16_block/2(State_theta_pll_GFL_16_38575), i_q_GFL_16_block/4(State_theta_pll_GFL_16_9c98e), d_Phipll_GFL_16_block/2(State_theta_pll_GFL_16_31350), d_Psi_d_GFL_16_block/2(State_theta_pll_GFL_16_f203b), d_Idv_GFL_16_block/9(State_theta_pll_GFL_16_10000), d_Iqv_GFL_16_block/9(State_theta_pll_GFL_16_db814), i_d_GFL_16_block/2(State_theta_pll_GFL_16_be048), i_d_GFL_16_block/4(State_theta_pll_GFL_16_4b91a)
  v_d_GFL_16/1 -> d_i_gd_GFL_16_block/1(Input_v_d_GFL_16_f719a), d_i_gq_GFL_16_block/12(Input_v_d_GFL_16_f3aaf), d_V_dc_GFL_16_block/14(Input_v_d_GFL_16_3e044), d_V_dc_GFL_16_block/20(Input_v_d_GFL_16_7444a), d_V_dc_GFL_16_block/31(Input_v_d_GFL_16_2c47b), d_theta_pll_GFL_16_block/1(Input_v_d_GFL_16_c3931), d_V_dc_GFL_16_block/38(Input_v_d_GFL_16_7f1f3), d_Phi_gd_GFL_16_block/1(Input_v_d_GFL_16_9b711), d_V_dc_GFL_16_block/5(Input_v_d_GFL_16_6e82b), d_Phi_gd_GFL_16_block/7(Input_v_d_GFL_16_a7f85), d_i_gq_GFL_16_block/7(Input_v_d_GFL_16_21396), d_Idv_GFL_16_block/2(Input_v_d_GFL_16_7be83), d_Idv_GFL_16_block/6(Input_v_d_GFL_16_fb423), d_Iqv_GFL_16_block/2(Input_v_d_GFL_16_a7d3d), d_Phi_gd_GFL_16_block/12(Input_v_d_GFL_16_1cbf7), d_Iqv_GFL_16_block/6(Input_v_d_GFL_16_3f07a), d_V_dc_GFL_16_block/26(Input_v_d_GFL_16_f6268), d_Phipll_GFL_16_block/1(Input_v_d_GFL_16_4ce7f), d_Phi_gc_GFL_16_block/7(Input_v_d_GFL_16_c77ca), d_Psi_d_GFL_16_block/1(Input_v_d_GFL_16_6aa9b), d_Psi_q_GFL_16_block/1(Input_v_d_GFL_16_3fb89), d_Phi_gb_GFL_16_block/1(Input_v_d_GFL_16_5796c), d_Phi_gc_GFL_16_block/2(Input_v_d_GFL_16_5298e), d_i_gq_GFL_16_block/1(Input_v_d_GFL_16_26005)
  v_q_GFL_16/1 -> d_i_gd_GFL_16_block/3(Input_v_q_GFL_16_05df1), d_i_gq_GFL_16_block/9(Input_v_q_GFL_16_5c00e), d_V_dc_GFL_16_block/7(Input_v_q_GFL_16_2d758), d_V_dc_GFL_16_block/16(Input_v_q_GFL_16_384ed), d_V_dc_GFL_16_block/28(Input_v_q_GFL_16_a04ae), d_V_dc_GFL_16_block/33(Input_v_q_GFL_16_01629), d_V_dc_GFL_16_block/40(Input_v_q_GFL_16_dfa59), d_theta_pll_GFL_16_block/3(Input_v_q_GFL_16_f8c47), d_Phi_gd_GFL_16_block/3(Input_v_q_GFL_16_c9e4f), d_Phi_gd_GFL_16_block/9(Input_v_q_GFL_16_d5137), d_i_gq_GFL_16_block/14(Input_v_q_GFL_16_4d2d7), d_Iqv_GFL_16_block/4(Input_v_q_GFL_16_c2908), d_Phi_gd_GFL_16_block/14(Input_v_q_GFL_16_69c8c), d_i_gq_GFL_16_block/3(Input_v_q_GFL_16_f5e00), d_V_dc_GFL_16_block/22(Input_v_q_GFL_16_9ba49), d_Idv_GFL_16_block/4(Input_v_q_GFL_16_b65e9), d_Idv_GFL_16_block/8(Input_v_q_GFL_16_07e38), d_Iqv_GFL_16_block/8(Input_v_q_GFL_16_1ea2b), d_Phipll_GFL_16_block/3(Input_v_q_GFL_16_4b778), d_Phi_gc_GFL_16_block/4(Input_v_q_GFL_16_b8cf3), d_Phi_gc_GFL_16_block/9(Input_v_q_GFL_16_61e16), d_Psi_d_GFL_16_block/3(Input_v_q_GFL_16_54a29), d_Psi_q_GFL_16_block/3(Input_v_q_GFL_16_21710), d_Phi_gb_GFL_16_block/3(Input_v_q_GFL_16_58470)
  d_Phi_gc_GFL_16_block/1(Blockout_d_Phi_gc_GFL_16_21552) -> Phi_gc_GFL_16/1
  d_Phi_gb_GFL_16_block/1(Blockout_d_Phi_gb_GFL_16_e3dc3) -> Phi_gb_GFL_16/1
  d_Phi_ga_GFL_16_block/1(Blockout_d_Phi_ga_GFL_16_6a1ed) -> Phi_ga_GFL_16/1
  d_Phipll_GFL_16_block/1(Blockout_d_Phipll_GFL_16_c41f9) -> Phipll_GFL_16/1
  d_V_dc_GFL_16_block/1(Blockout_d_V_dc_GFL_16_8cb25) -> V_dc_GFL_16/1
  Phi_gc_GFL_16/1 -> d_Phi_gd_GFL_16_block/16(State_Phi_gc_GFL_16_a3666), d_i_gq_GFL_16_block/16(State_Phi_gc_GFL_16_ded18), d_V_dc_GFL_16_block/35(State_Phi_gc_GFL_16_8b374)
  Phi_gb_GFL_16/1 -> d_V_dc_GFL_16_block/13(State_Phi_gb_GFL_16_76ba1), d_i_gd_GFL_16_block/9(State_Phi_gb_GFL_16_1e17f)
  Psi_d_GFL_16/1 -> d_Psi_d_GFL_16_block/5(State_Psi_d_GFL_16_eadb2), d_Idv_GFL_16_block/10(State_Psi_d_GFL_16_8afd7)
  Iqv_GFL_16/1 -> d_V_dc_GFL_16_block/24(State_Iqv_GFL_16_9facd), d_Iqv_GFL_16_block/1(State_Iqv_GFL_16_85f35), d_i_gq_GFL_16_block/5(State_Iqv_GFL_16_fce4f), d_Phi_gd_GFL_16_block/5(State_Iqv_GFL_16_6ee1c)

== system IEEE14_case/GFL_17 ==
  v_d_GFL_17 : Inport
  v_q_GFL_17 : Inport  Port=2
  i_dc_GFL_17 : Inport  Port=3
  Idv_GFL_17 : Integrator  InitialCondition=-1.3656732656210737e-20
  Iqv_GFL_17 : Integrator  InitialCondition=211.55079180000052
  Phi_ga_GFL_17 : Integrator  InitialCondition=14.491868689819446
  Phi_gb_GFL_17 : Integrator  InitialCondition=4.732187253972927
  Phi_gc_GFL_17 : Integrator  InitialCondition=-214.27992490452453
  Phi_gd_GFL_17 : Integrator  InitialCondition=-0.9464374507946149
  Phipll_GFL_17 : Integrator  InitialCondition=1.2551772502334691e-21
  Psi_d_GFL_17 : Integrator  InitialCondition=-2.8623909351197677e-22
  Psi_q_GFL_17 : Integrator  InitialCondition=21.15507918000005
  V_dc_GFL_17 : Integrator  InitialCondition=708.1423290583741
  d_Idv_GFL_17_block : Subsystem
  d_Iqv_GFL_17_block : Subsystem
  d_Phi_ga_GFL_17_block : Subsystem
  d_Phi_gb_GFL_17_block : Subsystem
  d_Phi_gc_GFL_17_block : Subsystem
  d_Phi_gd_GFL_17_block : Subsystem
  d_Phipll_GFL_17_block : Subsystem
  d_Psi_d_GFL_17_block : Subsystem
  d_Psi_q_GFL_17_block : Subsystem
  d_V_dc_GFL_17_block : Subsystem
  d_i_gd_GFL_17_block : Subsystem
  d_i_gq_GFL_17_block : Subsystem
  d_theta_pll_GFL_17_block : Subsystem
  e_dc_GFL_17_block : Subsystem
  i_d_GFL_17_block : Subsystem
  i_gd_GFL_17 : Integrator  InitialCondition=13.645665522619444
  i_gq_GFL_17 : Integrator  InitialCondition=-2.7291331045240073
  i_q_GFL_17_block : Subsystem
  theta_pll_GFL_17 : Integrator  InitialCondition=0.12690895074286768
  i_d_GFL_17 : Outport
  i_q_GFL_17 : Outport  Port=2
  e_dc_GFL_17 : Outport  Port=3
  wires:
  Phi_ga_GFL_17/1 -> d_V_dc_GFL_17_block/11(State_Phi_ga_GFL_17_55e9b), d_i_gd_GFL_17_block/7(State_Phi_ga_GFL_17_11b44), d_Phi_gb_GFL_17_block/7(State_Phi_ga_GFL_17_0e94a)
  Phi_gb_GFL_17/1 -> d_V_dc_GFL_17_block/13(State_Phi_gb_GFL_17_a014d), d_i_gd_GFL_17_block/9(State_Phi_gb_GFL_17_45475)
  i_dc_GFL_17/1 -> d_V_dc_GFL_17_block/2(Input_i_dc_GFL_17_b2e3f)
  theta_pll_GFL_17/1 -> d_i_gd_GFL_17_block/2(State_theta_pll_GFL_17_c766c), d_i_gq_GFL_17_block/2(State_theta_pll_GFL_17_54061), d_i_gq_GFL_17_block/8(State_theta_pll_GFL_17_ade9f), d_i_gq_GFL_17_block/13(State_theta_pll_GFL_17_c1a20), d_V_dc_GFL_17_block/6(State_theta_pll_GFL_17_ce4a2), d_V_dc_GFL_17_block/8(State_theta_pll_GFL_17_4a347), d_V_dc_GFL_17_block/17(State_theta_pll_GFL_17_bd8c4), d_V_dc_GFL_17_block/15(State_theta_pll_GFL_17_9bdeb), d_V_dc_GFL_17_block/27(State_theta_pll_GFL_17_8f50d), d_V_dc_GFL_17_block/34(State_theta_pll_GFL_17_c2799), d_V_dc_GFL_17_block/29(State_theta_pll_GFL_17_b2824), d_i_gq_GFL_17_block/15(State_theta_pll_GFL_17_d56bc), d_theta_pll_GFL_17_block/2(State_theta_pll_GFL_17_4c41d), d_theta_pll_GFL_17_block/4(State_theta_pll_GFL_17_280fb), d_Phi_gb_GFL_17_block/2(State_theta_pll_GFL_17_d7184), d_i_gd_GFL_17_block/4(State_theta_pll_GFL_17_748be), d_V_dc_GFL_17_block/41(State_theta_pll_GFL_17_03f60), d_V_dc_GFL_17_block/39(State_theta_pll_GFL_17_12fff), d_Phi_gd_GFL_17_block/2(State_theta_pll_GFL_17_b7930), d_Phi_gd_GFL_17_block/4(State_theta_pll_GFL_17_4bbd3), d_Phi_gd_GFL_17_block/8(State_theta_pll_GFL_17_40a47), d_Phi_gd_GFL_17_block/10(State_theta_pll_GFL_17_774b0), d_Phi_gd_GFL_17_block/15(State_theta_pll_GFL_17_61b54), d_Phi_gd_GFL_17_block/13(State_theta_pll_GFL_17_735fc), d_V_dc_GFL_17_block/23(State_theta_pll_GFL_17_4c26e), d_Idv_GFL_17_block/3(State_theta_pll_GFL_17_9e194), d_Idv_GFL_17_block/5(State_theta_pll_GFL_17_44aa2), d_Idv_GFL_17_block/7(State_theta_pll_GFL_17_82810), d_Iqv_GFL_17_block/3(State_theta_pll_GFL_17_38143), d_i_gq_GFL_17_block/4(State_theta_pll_GFL_17_ae1e4), d_Iqv_GFL_17_block/9(State_theta_pll_GFL_17_b5422), d_Idv_GFL_17_block/9(State_theta_pll_GFL_17_629fa), d_Iqv_GFL_17_block/5(State_theta_pll_GFL_17_2973d), d_V_dc_GFL_17_block/32(State_theta_pll_GFL_17_43992), d_i_gq_GFL_17_block/10(State_theta_pll_GFL_17_5e05a), d_Iqv_GFL_17_block/7(State_theta_pll_GFL_17_aa9de), d_V_dc_GFL_17_block/21(State_theta_pll_GFL_17_e2101), d_Phipll_GFL_17_block/2(State_theta_pll_GFL_17_b324e), d_Phipll_GFL_17_block/4(State_theta_pll_GFL_17_05e65), d_Phi_gc_GFL_17_block/3(State_theta_pll_GFL_17_39a31), d_Phi_gc_GFL_17_block/10(State_theta_pll_GFL_17_44558), d_Psi_d_GFL_17_block/2(State_theta_pll_GFL_17_99832), d_Psi_d_GFL_17_block/4(State_theta_pll_GFL_17_a4bf5), d_Psi_q_GFL_17_block/2(State_theta_pll_GFL_17_ec146), d_Psi_q_GFL_17_block/4(State_theta_pll_GFL_17_743ba), i_d_GFL_17_block/2(State_theta_pll_GFL_17_d2c5b), i_d_GFL_17_block/4(State_theta_pll_GFL_17_5024c), i_q_GFL_17_block/2(State_theta_pll_GFL_17_da001), i_q_GFL_17_block/4(State_theta_pll_GFL_17_5726e), d_Phi_gc_GFL_17_block/5(State_theta_pll_GFL_17_1661f), d_Phi_gb_GFL_17_block/4(State_theta_pll_GFL_17_d1250), d_Phi_gc_GFL_17_block/8(State_theta_pll_GFL_17_c6e4e)
  d_Phi_ga_GFL_17_block/1(Blockout_d_Phi_ga_GFL_17_7246c) -> Phi_ga_GFL_17/1
  d_Idv_GFL_17_block/1(Blockout_d_Idv_GFL_17_3c079) -> Idv_GFL_17/1
  d_Iqv_GFL_17_block/1(Blockout_d_Iqv_GFL_17_0648b) -> Iqv_GFL_17/1
  d_Phipll_GFL_17_block/1(Blockout_d_Phipll_GFL_17_3d5a8) -> Phipll_GFL_17/1
  d_i_gq_GFL_17_block/1(Blockout_d_i_gq_GFL_17_a2246) -> i_gq_GFL_17/1
  Phipll_GFL_17/1 -> d_theta_pll_GFL_17_block/5(State_Phipll_GFL_17_89cae)
  d_Psi_q_GFL_17_block/1(Blockout_d_Psi_q_GFL_17_9f89a) -> Psi_q_GFL_17/1
  i_d_GFL_17_block/1(Blockout_i_d_GFL_17_3e529) -> i_d_GFL_17/1
  V_dc_GFL_17/1 -> d_V_dc_GFL_17_block/10(State_V_dc_GFL_17_1c4d8), d_V_dc_GFL_17_block/42(State_V_dc_GFL_17_4d001), d_V_dc_GFL_17_block/1(State_V_dc_GFL_17_61ba6), d_Phi_gb_GFL_17_block/6(State_V_dc_GFL_17_71b96), d_i_gd_GFL_17_block/6(State_V_dc_GFL_17_0edd3), e_dc_GFL_17_block/1(State_V_dc_GFL_17_df3ee), d_Phi_ga_GFL_17_block/1(State_V_dc_GFL_17_b46a6)
  i_gq_GFL_17/1 -> d_Phi_gd_GFL_17_block/17(State_i_gq_GFL_17_3bf40), d_i_gq_GFL_17_block/17(State_i_gq_GFL_17_272c2), d_V_dc_GFL_17_block/30(State_i_gq_GFL_17_e224f), d_V_dc_GFL_17_block/4(State_i_gq_GFL_17_13802), d_i_gq_GFL_17_block/11(State_i_gq_GFL_17_952ec), d_V_dc_GFL_17_block/36(State_i_gq_GFL_17_7fe40), d_V_dc_GFL_17_block/18(State_i_gq_GFL_17_f2530), d_Phi_gd_GFL_17_block/11(State_i_gq_GFL_17_b900e), d_i_gq_GFL_17_block/19(State_i_gq_GFL_17_921b2), d_Phi_gc_GFL_17_block/6(State_i_gq_GFL_17_83f75), i_q_GFL_17_block/3(State_i_gq_GFL_17_4b654), i_d_GFL_17_block/3(State_i_gq_GFL_17_23567)
  e_dc_GFL_17_block/1(Blockout_e_dc_GFL_17_f966e) -> e_dc_GFL_17/1
  i_q_GFL_17_block/1(Blockout_i_q_GFL_17_34d19) -> i_q_GFL_17/1
  Idv_GFL_17/1 -> d_V_dc_GFL_17_block/9(State_Idv_GFL_17_e3537), d_Idv_GFL_17_block/1(State_Idv_GFL_17_dbb4f), d_i_gd_GFL_17_block/5(State_Idv_GFL_17_31090), d_Phi_gb_GFL_17_block/5(State_Idv_GFL_17_5ec1c)
  d_i_gd_GFL_17_block/1(Blockout_d_i_gd_GFL_17_06168) -> i_gd_GFL_17/1
  d_Psi_d_GFL_17_block/1(Blockout_d_Psi_d_GFL_17_6e508) -> Psi_d_GFL_17/1
  d_Phi_gd_GFL_17_block/1(Blockout_d_Phi_gd_GFL_17_94f94) -> Phi_gd_GFL_17/1
  d_Phi_gc_GFL_17_block/1(Blockout_d_Phi_gc_GFL_17_224f3) -> Phi_gc_GFL_17/1
  d_Phi_gb_GFL_17_block/1(Blockout_d_Phi_gb_GFL_17_572a8) -> Phi_gb_GFL_17/1
  d_V_dc_GFL_17_block/1(Blockout_d_V_dc_GFL_17_353cb) -> V_dc_GFL_17/1
  Psi_d_GFL_17/1 -> d_Psi_d_GFL_17_block/5(State_Psi_d_GFL_17_04c08), d_Idv_GFL_17_block/10(State_Psi_d_GFL_17_f48a9)
  Psi_q_GFL_17/1 -> d_Psi_q_GFL_17_block/5(State_Psi_q_GFL_17_1cfcb), d_Iqv_GFL_17_block/10(State_Psi_q_GFL_17_98c01)
  Phi_gc_GFL_17/1 -> d_Phi_gd_GFL_17_block/16(State_Phi_gc_GFL_17_57f27), d_i_gq_GFL_17_block/16(State_Phi_gc_GFL_17_446f2), d_V_dc_GFL_17_block/35(State_Phi_gc_GFL_17_ca63d)
  v_q_GFL_17/1 -> d_i_gd_GFL_17_block/3(Input_v_q_GFL_17_15e66), d_i_gq_GFL_17_block/9(Input_v_q_GFL_17_19e6b), d_i_gq_GFL_17_block/14(Input_v_q_GFL_17_9c3f0), d_V_dc_GFL_17_block/16(Input_v_q_GFL_17_0e6b7), d_V_dc_GFL_17_block/33(Input_v_q_GFL_17_ff76b), d_theta_pll_GFL_17_block/3(Input_v_q_GFL_17_afffd), d_Phi_gb_GFL_17_block/3(Input_v_q_GFL_17_c3fa8), d_Idv_GFL_17_block/8(Input_v_q_GFL_17_30fdf), d_V_dc_GFL_17_block/7(Input_v_q_GFL_17_2aff7), d_Phi_gd_GFL_17_block/14(Input_v_q_GFL_17_f280b), d_Iqv_GFL_17_block/8(Input_v_q_GFL_17_37f0a), d_Idv_GFL_17_block/4(Input_v_q_GFL_17_e3e51), d_V_dc_GFL_17_block/22(Input_v_q_GFL_17_b68cc), d_Phi_gd_GFL_17_block/3(Input_v_q_GFL_17_e089c), d_Iqv_GFL_17_block/4(Input_v_q_GFL_17_45d80), d_i_gq_GFL_17_block/3(Input_v_q_GFL_17_9adff), d_Phi_gd_GFL_17_block/9(Input_v_q_GFL_17_bac0f), d_Phi_gc_GFL_17_block/9(Input_v_q_GFL_17_b7629), d_Psi_d_GFL_17_block/3(Input_v_q_GFL_17_2c18f), d_Psi_q_GFL_17_block/3(Input_v_q_GFL_17_699cf), d_Phi_gc_GFL_17_block/4(Input_v_q_GFL_17_9c131), d_Phipll_GFL_17_block/3(Input_v_q_GFL_17_cfbee), d_V_dc_GFL_17_block/28(Input_v_q_GFL_17_959f8), d_V_dc_GFL_17_block/40(Input_v_q_GFL_17_0295a)
  Phi_gd_GFL_17/1 -> d_V_dc_GFL_17_block/37(State_Phi_gd_GFL_17_8444d), d_i_gq_GFL_17_block/18(State_Phi_gd_GFL_17_5b911)
  i_gd_GFL_17/1 -> d_V_dc_GFL_17_block/25(State_i_gd_GFL_17_097e8), d_i_gd_GFL_17_block/10(State_i_gd_GFL_17_d59fc), d_V_dc_GFL_17_block/19(State_i_gd_GFL_17_ee33a), d_V_dc_GFL_17_block/12(State_i_gd_GFL_17_9e4d0), d_Phi_gd_GFL_17_block/6(State_i_gd_GFL_17_cda7b), d_i_gd_GFL_17_block/8(State_i_gd_GFL_17_ac7fa), d_i_gq_GFL_17_block/6(State_i_gd_GFL_17_be3a3), d_V_dc_GFL_17_block/3(State_i_gd_GFL_17_c8e95), d_Phi_gc_GFL_17_block/1(State_i_gd_GFL_17_74615), i_q_GFL_17_block/1(State_i_gd_GFL_17_b074d), d_Phi_gb_GFL_17_block/8(State_i_gd_GFL_17_f44e4), i_d_GFL_17_block/1(State_i_gd_GFL_17_ef23a)
  v_d_GFL_17/1 -> d_i_gq_GFL_17_block/1(Input_v_d_GFL_17_26746), d_i_gq_GFL_17_block/7(Input_v_d_GFL_17_c62dd), d_i_gq_GFL_17_block/12(Input_v_d_GFL_17_a9001), d_V_dc_GFL_17_block/5(Input_v_d_GFL_17_69f5b), d_V_dc_GFL_17_block/14(Input_v_d_GFL_17_85bd5), d_V_dc_GFL_17_block/26(Input_v_d_GFL_17_4b47a), d_V_dc_GFL_17_block/31(Input_v_d_GFL_17_cb6ad), d_V_dc_GFL_17_block/38(Input_v_d_GFL_17_ffaea), d_theta_pll_GFL_17_block/1(Input_v_d_GFL_17_db4bf), d_Phi_gb_GFL_17_block/1(Input_v_d_GFL_17_375e3), d_i_gd_GFL_17_block/1(Input_v_d_GFL_17_f609b), d_Phi_gd_GFL_17_block/12(Input_v_d_GFL_17_a70b9), d_Idv_GFL_17_block/2(Input_v_d_GFL_17_0e53b), d_V_dc_GFL_17_block/20(Input_v_d_GFL_17_e38bd), d_Phi_gd_GFL_17_block/7(Input_v_d_GFL_17_2017d), d_Phi_gd_GFL_17_block/1(Input_v_d_GFL_17_5111b), d_Idv_GFL_17_block/6(Input_v_d_GFL_17_235ef), d_Iqv_GFL_17_block/2(Input_v_d_GFL_17_2ae22), d_Iqv_GFL_17_block/6(Input_v_d_GFL_17_ad61a), d_Phipll_GFL_17_block/1(Input_v_d_GFL_17_09fe8), d_Phi_gc_GFL_17_block/2(Input_v_d_GFL_17_9c85a), d_Phi_gc_GFL_17_block/7(Input_v_d_GFL_17_ad008), d_Psi_q_GFL_17_block/1(Input_v_d_GFL_17_9db94), d_Psi_d_GFL_17_block/1(Input_v_d_GFL_17_e6869)
  Iqv_GFL_17/1 -> d_V_dc_GFL_17_block/24(State_Iqv_GFL_17_27d19), d_Iqv_GFL_17_block/1(State_Iqv_GFL_17_66272), d_i_gq_GFL_17_block/5(State_Iqv_GFL_17_7539a), d_Phi_gd_GFL_17_block/5(State_Iqv_GFL_17_1b144)
  d_theta_pll_GFL_17_block/1(Blockout_d_theta_pll_GFL_17_04ce6) -> theta_pll_GFL_17/1

== system IEEE14_case/GFL_18 ==
  v_d_GFL_18 : Inport
  v_q_GFL_18 : Inport  Port=2
  i_dc_GFL_18 : Inport  Port=3
  Idv_GFL_18 : Integrator  InitialCondition=-1.466404611278312e-19
  Iqv_GFL_18 : Integrator  InitialCondition=212.0998158000034
  Phi_ga_GFL_18 : Integrator  InitialCondition=14.458742747279334
  Phi_gb_GFL_18 : Integrator  InitialCondition=4.719937906347706
  Phi_gc_GFL_18 : Integrator  InitialCondition=-214.82188449682
  Phi_gd_GFL_18 : Integrator  InitialCondition=-0.9439875812697851
  Phipll_GFL_18 : Integrator  InitialCondition=-8.934824614593479e-20
  Psi_d_GFL_18 : Integrator  InitialCondition=5.7057889991864425e-21
  Psi_q_GFL_18 : Integrator  InitialCondition=21.209981580000342
  V_dc_GFL_18 : Integrator  InitialCondition=708.1002304640865
  d_Idv_GFL_18_block : Subsystem
  d_Iqv_GFL_18_block : Subsystem
  d_Phi_ga_GFL_18_block : Subsystem
  d_Phi_gb_GFL_18_block : Subsystem
  d_Phi_gc_GFL_18_block : Subsystem
  d_Phi_gd_GFL_18_block : Subsystem
  d_Phipll_GFL_18_block : Subsystem
  d_Psi_d_GFL_18_block : Subsystem
  d_Psi_q_GFL_18_block : Subsystem
  d_V_dc_GFL_18_block : Subsystem
  d_i_gd_GFL_18_block : Subsystem
  d_i_gq_GFL_18_block : Subsystem
  d_theta_pll_GFL_18_block : Subsystem
  e_dc_GFL_18_block : Subsystem
  i_d_GFL_18_block : Subsystem
  i_gd_GFL_18 : Integrator  InitialCondition=13.610343484079321
  i_gq_GFL_18 : Integrator  InitialCondition=-2.7220686968165864
  i_q_GFL_18_block : Subsystem
  theta_pll_GFL_18 : Integrator  InitialCondition=0.14526242230633082
  i_d_GFL_18 : Outport
  i_q_GFL_18 : Outport  Port=2
  e_dc_GFL_18 : Outport  Port=3
  wires:
  Phipll_GFL_18/1 -> d_theta_pll_GFL_18_block/5(State_Phipll_GFL_18_8c922)
  i_gq_GFL_18/1 -> d_i_gq_GFL_18_block/11(State_i_gq_GFL_18_16534), d_V_dc_GFL_18_block/4(State_i_gq_GFL_18_6e18c), d_V_dc_GFL_18_block/30(State_i_gq_GFL_18_75421), d_V_dc_GFL_18_block/18(State_i_gq_GFL_18_13b92), d_i_gq_GFL_18_block/19(State_i_gq_GFL_18_b9a26), d_i_gq_GFL_18_block/17(State_i_gq_GFL_18_9395d), d_Phi_gd_GFL_18_block/17(State_i_gq_GFL_18_464a8), d_V_dc_GFL_18_block/36(State_i_gq_GFL_18_e5033), d_Phi_gc_GFL_18_block/6(State_i_gq_GFL_18_622c8), d_Phi_gd_GFL_18_block/11(State_i_gq_GFL_18_21998), i_d_GFL_18_block/3(State_i_gq_GFL_18_5a399), i_q_GFL_18_block/3(State_i_gq_GFL_18_d9fa7)
  i_gd_GFL_18/1 -> d_i_gq_GFL_18_block/6(State_i_gd_GFL_18_52805), d_Phi_gd_GFL_18_block/6(State_i_gd_GFL_18_2dd77), d_V_dc_GFL_18_block/25(State_i_gd_GFL_18_beff4), d_V_dc_GFL_18_block/12(State_i_gd_GFL_18_1b00f), d_V_dc_GFL_18_block/19(State_i_gd_GFL_18_b4d7b), d_V_dc_GFL_18_block/3(State_i_gd_GFL_18_3d6da), d_Phi_gb_GFL_18_block/8(State_i_gd_GFL_18_25876), d_i_gd_GFL_18_block/8(State_i_gd_GFL_18_d4705), d_i_gd_GFL_18_block/10(State_i_gd_GFL_18_ac69d), i_q_GFL_18_block/1(State_i_gd_GFL_18_76c93), i_d_GFL_18_block/1(State_i_gd_GFL_18_d192a), d_Phi_gc_GFL_18_block/1(State_i_gd_GFL_18_5899c)
  Iqv_GFL_18/1 -> d_V_dc_GFL_18_block/24(State_Iqv_GFL_18_42d53), d_Iqv_GFL_18_block/1(State_Iqv_GFL_18_dba96), d_i_gq_GFL_18_block/5(State_Iqv_GFL_18_30b1b), d_Phi_gd_GFL_18_block/5(State_Iqv_GFL_18_70c7a)
  v_d_GFL_18/1 -> d_i_gd_GFL_18_block/1(Input_v_d_GFL_18_95c19), d_i_gq_GFL_18_block/1(Input_v_d_GFL_18_6f882), d_i_gq_GFL_18_block/7(Input_v_d_GFL_18_7a2d9), d_i_gq_GFL_18_block/12(Input_v_d_GFL_18_2cf8e), d_V_dc_GFL_18_block/5(Input_v_d_GFL_18_701fe), d_V_dc_GFL_18_block/14(Input_v_d_GFL_18_fe6e3), d_V_dc_GFL_18_block/20(Input_v_d_GFL_18_90dae), d_V_dc_GFL_18_block/31(Input_v_d_GFL_18_a399d), d_V_dc_GFL_18_block/38(Input_v_d_GFL_18_04e5f), d_theta_pll_GFL_18_block/1(Input_v_d_GFL_18_139e6), d_Phi_gb_GFL_18_block/1(Input_v_d_GFL_18_d4937), d_Phi_gd_GFL_18_block/7(Input_v_d_GFL_18_27679), d_Phi_gd_GFL_18_block/12(Input_v_d_GFL_18_ab6ff), d_Idv_GFL_18_block/6(Input_v_d_GFL_18_0ae0e), d_V_dc_GFL_18_block/26(Input_v_d_GFL_18_feb25), d_Phi_gd_GFL_18_block/1(Input_v_d_GFL_18_11d9f), d_Idv_GFL_18_block/2(Input_v_d_GFL_18_10cbd), d_Iqv_GFL_18_block/2(Input_v_d_GFL_18_b6341), d_Phipll_GFL_18_block/1(Input_v_d_GFL_18_58041), d_Phi_gc_GFL_18_block/2(Input_v_d_GFL_18_02ef3), d_Phi_gc_GFL_18_block/7(Input_v_d_GFL_18_79bfc), d_Psi_d_GFL_18_block/1(Input_v_d_GFL_18_5d979), d_Psi_q_GFL_18_block/1(Input_v_d_GFL_18_32a52), d_Iqv_GFL_18_block/6(Input_v_d_GFL_18_59aa3)
  d_Phipll_GFL_18_block/1(Blockout_d_Phipll_GFL_18_24764) -> Phipll_GFL_18/1
  d_Idv_GFL_18_block/1(Blockout_d_Idv_GFL_18_15e6a) -> Idv_GFL_18/1
  d_theta_pll_GFL_18_block/1(Blockout_d_theta_pll_GFL_18_8cdeb) -> theta_pll_GFL_18/1
  d_Phi_gc_GFL_18_block/1(Blockout_d_Phi_gc_GFL_18_de35a) -> Phi_gc_GFL_18/1
  Phi_ga_GFL_18/1 -> d_V_dc_GFL_18_block/11(State_Phi_ga_GFL_18_22e90), d_i_gd_GFL_18_block/7(State_Phi_ga_GFL_18_805dd), d_Phi_gb_GFL_18_block/7(State_Phi_ga_GFL_18_0803b)
  theta_pll_GFL_18/1 -> d_i_gq_GFL_18_block/8(State_theta_pll_GFL_18_d5076), d_i_gq_GFL_18_block/10(State_theta_pll_GFL_18_46ba7), d_V_dc_GFL_18_block/6(State_theta_pll_GFL_18_eb734), d_V_dc_GFL_18_block/8(State_theta_pll_GFL_18_1f369), d_V_dc_GFL_18_block/23(State_theta_pll_GFL_18_b331e), d_V_dc_GFL_18_block/34(State_theta_pll_GFL_18_74cd7), d_V_dc_GFL_18_block/27(State_theta_pll_GFL_18_9b374), d_i_gq_GFL_18_block/13(State_theta_pll_GFL_18_ab8d9), d_V_dc_GFL_18_block/39(State_theta_pll_GFL_18_ec64f), d_V_dc_GFL_18_block/41(State_theta_pll_GFL_18_6eb5f), d_theta_pll_GFL_18_block/2(State_theta_pll_GFL_18_5174e), d_Phi_gb_GFL_18_block/2(State_theta_pll_GFL_18_76645), d_Phi_gb_GFL_18_block/4(State_theta_pll_GFL_18_60c54), d_Phi_gd_GFL_18_block/8(State_theta_pll_GFL_18_40df2), d_Phi_gd_GFL_18_block/10(State_theta_pll_GFL_18_8d0fd), d_i_gq_GFL_18_block/4(State_theta_pll_GFL_18_9acfa), d_Phi_gd_GFL_18_block/15(State_theta_pll_GFL_18_ec069), d_V_dc_GFL_18_block/15(State_theta_pll_GFL_18_cc95e), d_V_dc_GFL_18_block/29(State_theta_pll_GFL_18_70e0e), d_Idv_GFL_18_block/5(State_theta_pll_GFL_18_96f6a), d_Idv_GFL_18_block/7(State_theta_pll_GFL_18_4866f), d_Idv_GFL_18_block/9(State_theta_pll_GFL_18_af8c5), d_i_gd_GFL_18_block/4(State_theta_pll_GFL_18_bdc92), d_Iqv_GFL_18_block/5(State_theta_pll_GFL_18_b687b), d_theta_pll_GFL_18_block/4(State_theta_pll_GFL_18_62af6), d_Iqv_GFL_18_block/7(State_theta_pll_GFL_18_7a1d2), d_Iqv_GFL_18_block/9(State_theta_pll_GFL_18_15ee8), d_i_gd_GFL_18_block/2(State_theta_pll_GFL_18_c6cb4), d_Phi_gd_GFL_18_block/13(State_theta_pll_GFL_18_77a50), d_V_dc_GFL_18_block/17(State_theta_pll_GFL_18_69e87), d_V_dc_GFL_18_block/21(State_theta_pll_GFL_18_03dba), d_V_dc_GFL_18_block/32(State_theta_pll_GFL_18_bb071), d_Phi_gd_GFL_18_block/4(State_theta_pll_GFL_18_7f5d8), d_Iqv_GFL_18_block/3(State_theta_pll_GFL_18_8f911), d_Idv_GFL_18_block/3(State_theta_pll_GFL_18_4128c), d_i_gq_GFL_18_block/15(State_theta_pll_GFL_18_cabe0), d_Phi_gd_GFL_18_block/2(State_theta_pll_GFL_18_6022b), d_Phipll_GFL_18_block/2(State_theta_pll_GFL_18_676c3), d_Phipll_GFL_18_block/4(State_theta_pll_GFL_18_5129b), d_Phi_gc_GFL_18_block/3(State_theta_pll_GFL_18_ce778), d_Phi_gc_GFL_18_block/5(State_theta_pll_GFL_18_3fc4b), d_Phi_gc_GFL_18_block/8(State_theta_pll_GFL_18_d8932), d_Psi_d_GFL_18_block/2(State_theta_pll_GFL_18_3c1b0), d_Psi_d_GFL_18_block/4(State_theta_pll_GFL_18_19ef9), d_Psi_q_GFL_18_block/2(State_theta_pll_GFL_18_7c914), d_Psi_q_GFL_18_block/4(State_theta_pll_GFL_18_501c5), i_d_GFL_18_block/2(State_theta_pll_GFL_18_bcee7), i_d_GFL_18_block/4(State_theta_pll_GFL_18_13217), i_q_GFL_18_block/2(State_theta_pll_GFL_18_ffcf5), i_q_GFL_18_block/4(State_theta_pll_GFL_18_e08cb), d_Phi_gc_GFL_18_block/10(State_theta_pll_GFL_18_57f3c), d_i_gq_GFL_18_block/2(State_theta_pll_GFL_18_750f2)
  i_dc_GFL_18/1 -> d_V_dc_GFL_18_block/2(Input_i_dc_GFL_18_c4cfa)
  e_dc_GFL_18_block/1(Blockout_e_dc_GFL_18_f7b34) -> e_dc_GFL_18/1
  i_q_GFL_18_block/1(Blockout_i_q_GFL_18_d2cea) -> i_q_GFL_18/1
  Phi_gc_GFL_18/1 -> d_i_gq_GFL_18_block/16(State_Phi_gc_GFL_18_55584), d_Phi_gd_GFL_18_block/16(State_Phi_gc_GFL_18_ff2c0), d_V_dc_GFL_18_block/35(State_Phi_gc_GFL_18_41070)
  d_Phi_gb_GFL_18_block/1(Blockout_d_Phi_gb_GFL_18_4adfd) -> Phi_gb_GFL_18/1
  d_Iqv_GFL_18_block/1(Blockout_d_Iqv_GFL_18_c4d55) -> Iqv_GFL_18/1
  d_i_gd_GFL_18_block/1(Blockout_d_i_gd_GFL_18_28d76) -> i_gd_GFL_18/1
  Psi_q_GFL_18/1 -> d_Iqv_GFL_18_block/10(State_Psi_q_GFL_18_f1020), d_Psi_q_GFL_18_block/5(State_Psi_q_GFL_18_f8931)
  d_Psi_q_GFL_18_block/1(Blockout_d_Psi_q_GFL_18_327d3) -> Psi_q_GFL_18/1
  i_d_GFL_18_block/1(Blockout_i_d_GFL_18_7425f) -> i_d_GFL_18/1
  d_Psi_d_GFL_18_block/1(Blockout_d_Psi_d_GFL_18_ff813) -> Psi_d_GFL_18/1
  d_Phi_gd_GFL_18_block/1(Blockout_d_Phi_gd_GFL_18_10055) -> Phi_gd_GFL_18/1
  d_V_dc_GFL_18_block/1(Blockout_d_V_dc_GFL_18_00405) -> V_dc_GFL_18/1
  d_Phi_ga_GFL_18_block/1(Blockout_d_Phi_ga_GFL_18_9b191) -> Phi_ga_GFL_18/1
  Phi_gd_GFL_18/1 -> d_V_dc_GFL_18_block/37(State_Phi_gd_GFL_18_c93e4), d_i_gq_GFL_18_block/18(State_Phi_gd_GFL_18_5fde0)
  Psi_d_GFL_18/1 -> d_Psi_d_GFL_18_block/5(State_Psi_d_GFL_18_fcaf2), d_Idv_GFL_18_block/10(State_Psi_d_GFL_18_c430f)
  V_dc_GFL_18/1 -> d_V_dc_GFL_18_block/10(State_V_dc_GFL_18_c6017), d_Phi_gb_GFL_18_block/6(State_V_dc_GFL_18_6f965), d_i_gd_GFL_18_block/6(State_V_dc_GFL_18_90391), d_V_dc_GFL_18_block/42(State_V_dc_GFL_18_89786), d_V_dc_GFL_18_block/1(State_V_dc_GFL_18_3e782), e_dc_GFL_18_block/1(State_V_dc_GFL_18_327dd), d_Phi_ga_GFL_18_block/1(State_V_dc_GFL_18_2da35)
  Phi_gb_GFL_18/1 -> d_V_dc_GFL_18_block/13(State_Phi_gb_GFL_18_256d6), d_i_gd_GFL_18_block/9(State_Phi_gb_GFL_18_e630d)
  v_q_GFL_18/1 -> d_i_gq_GFL_18_block/9(Input_v_q_GFL_18_2227f), d_i_gq_GFL_18_block/14(Input_v_q_GFL_18_563cc), d_i_gd_GFL_18_block/3(Input_v_q_GFL_18_169b9), d_V_dc_GFL_18_block/7(Input_v_q_GFL_18_19803), d_V_dc_GFL_18_block/16(Input_v_q_GFL_18_6eb24), d_V_dc_GFL_18_block/28(Input_v_q_GFL_18_6d8da), d_V_dc_GFL_18_block/33(Input_v_q_GFL_18_349f9), d_Phi_gb_GFL_18_block/3(Input_v_q_GFL_18_3c3a2), d_Idv_GFL_18_block/4(Input_v_q_GFL_18_fc279), d_Idv_GFL_18_block/8(Input_v_q_GFL_18_9cb7b), d_V_dc_GFL_18_block/22(Input_v_q_GFL_18_518eb), d_Iqv_GFL_18_block/4(Input_v_q_GFL_18_86533), d_Phi_gd_GFL_18_block/14(Input_v_q_GFL_18_9cd88), d_V_dc_GFL_18_block/40(Input_v_q_GFL_18_9eebf), d_Iqv_GFL_18_block/8(Input_v_q_GFL_18_04b2f), d_Phi_gd_GFL_18_block/9(Input_v_q_GFL_18_95c1e), d_theta_pll_GFL_18_block/3(Input_v_q_GFL_18_f1179), d_Phi_gd_GFL_18_block/3(Input_v_q_GFL_18_3c803), d_i_gq_GFL_18_block/3(Input_v_q_GFL_18_fb235), d_Phipll_GFL_18_block/3(Input_v_q_GFL_18_0e9bd), d_Phi_gc_GFL_18_block/4(Input_v_q_GFL_18_ef739), d_Phi_gc_GFL_18_block/9(Input_v_q_GFL_18_a00d2), d_Psi_q_GFL_18_block/3(Input_v_q_GFL_18_f7ea8), d_Psi_d_GFL_18_block/3(Input_v_q_GFL_18_a3318)
  Idv_GFL_18/1 -> d_V_dc_GFL_18_block/9(State_Idv_GFL_18_a431e), d_Idv_GFL_18_block/1(State_Idv_GFL_18_af2bb), d_i_gd_GFL_18_block/5(State_Idv_GFL_18_f8d07), d_Phi_gb_GFL_18_block/5(State_Idv_GFL_18_7a112)
  d_i_gq_GFL_18_block/1(Blockout_d_i_gq_GFL_18_699bd) -> i_gq_GFL_18/1
